simulink model "EEBL_Scenario_01_cs"  (Simulink 7.6)
settings: Solver=ode5  SolverMode=SingleTasking  StartTime=0.0  StopTime=inf  FixedStep=1/100  RelTol=1e-3
PreLoadFcn:
  | check_NUTS_defined;
  | 
  | assignin('base',['model_closed_' bdroot],false);addpath('../includes_V2x');
InitFcn:
  | PreScanExperimentInitFcn(bdroot)
StopFcn:
  | PreScanExperimentStopFcn(bdroot)
undefined symbols (not defined in the file or in its folder): acceleration, actorID, actorType, DiscIntNeverNeededParam, GPS_alt, GPS_lat, GPS_long, intmax, lightBarInUse, messageID, publicVehicleType, rotZ, sireneInUse, trafficLightPriority, turnAdvice, velocity, x_ini_VRML, y_ini_VRML, yawRate, z_ini_VRML
libraries: simulink x58, PreScanSimulinkLibrary x12, simulink_extras x10, PreScanUsefulBlocks x6, simulink_need_slupdate x1
(part 2 of 10)

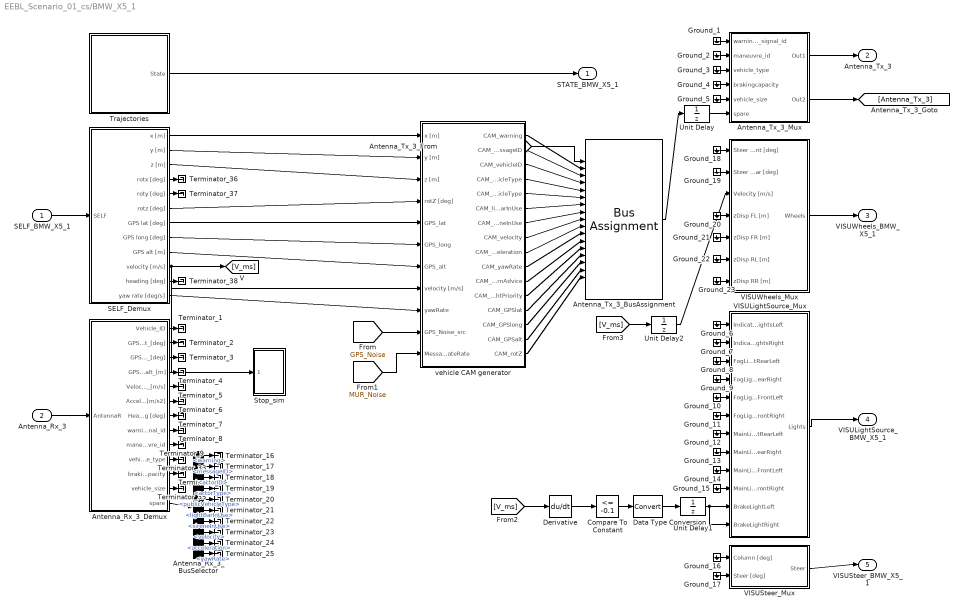
== system EEBL_Scenario_01_cs/BMW_X5_1 ==
  SELF_BMW_X5_1 : Inport  Tag=SELFInport
  Antenna_Rx_3 : Inport  Tag=AntennaRInport  Port=2
  Antenna_Rx_3_BusSelector : BusSelector  Tag=BusAntennaR  OutputSignals=warning,messageID,actorID,actorType,publicVehicleType,lightBarInUse,sireneInUse,velocity,acceleration,yawRate
  Antenna_Rx_3_Demux : Subsystem  Tag=DemuxAntennaR  mask(PreScan Demux Block:){Channel=1}
      settings: DeleteFcn=PreScanBlockDeleteFcn;
      mask Display:
      | fprintf('Channel: %d',Channel)
      | port_label('output', 1, 'Vehicle_ID')
      | port_label('output', 2, 'GPS Pos Lat [deg]')
      | port_label('output', 3, 'GPS Pos Long [deg]')
      | port_label('output', 4, 'GPS Pos Alt [m]')
      | port_label('output', 5, 'Velocity [m/s]')
      | port_label('output', 6, 'Acceleration [m/s2]')
      | port_label('output', 7, 'Heading [deg]')
      | port_label('output', 8, 'Warning signal ID')
      | port_label('output', 9, 'Maneuvre ID')
      | port_label('output', 10, 'Vehicle Type')
      | port_label('output', 11, 'Braking Capacity')
      | port_label('output', 12, 'Vehicle Size')
      | port_label('output', 13, 'Spare')
  Antenna_Tx_3_BusAssignment : BusAssignment  Tag=BusAntennaT  AssignedSignals=warning,messageID,actorID,actorType,publicVehicleType,lightBarInUse,sireneInUse,velocity,acceleration,yawRate,turnAdvice,trafficLightPriority,GPS_lat,GPS_long,GPS_alt,rotZ
  Antenna_Tx_3_Mux : Subsystem  Tag=MuxAntennaT  mask(PreScan Mux Block:){Channel=1, TimeStep=1/100}
      mask prompts: TimeStep "Time Step [s]"
      settings: DeleteFcn=PreScanBlockDeleteFcn;
      mask Display:
      | fprintf('Channel: %d',Channel)
      | port_label('input', 1, 'Warning signal ID')
      | port_label('input', 2, 'Maneuvre ID')
      | port_label('input', 3, 'Vehicle Type')
      | port_label('input', 4, 'Braking Capacity')
      | port_label('input', 5, 'Vehicle Size')
      | port_label('input', 6, 'spare')
  Compare To Constant : simulink/Logic and Bit Operations/Compare To Constant  SystemSampleTime=-1  relop=<=  const=-0.1  LogicOutDataTypeMode=boolean
  Data Type Conversion : DataTypeConversion
  Derivative : Derivative
  Ground_{1..23} (23 alike) : Ground
  SELF_Demux : Subsystem  Tag=DemuxSELF
      settings: DeleteFcn=PreScanBlockDeleteFcn;
      mask Type: PreScan Demux Block:
      mask Display:
      | port_label('output',1,'x [m]')
      | port_label('output',2,'y [m]')
      | port_label('output',3,'z [m]','texmode','on')
      | port_label('output',4,'Rotx [deg]','texmode','on')
      | port_label('output',5,'Roty [deg]','texmode','on')
      | port_label('output',6,'Rotz [deg]','texmode','on')
      | port_label('output',7,'GPS lat [deg]','texmode','on')
      | port_label('output',8,'GPS long [deg]','texmode','on')
      | port_label('output',9,'GPS alt [m]','texmode','on')
      | port_label('output',10,'Velocity [m/s]')
      | port_label('output',11,'Heading [deg]')
      | port_label('output',12,'Yaw rate [deg/s]')
  Stop_sim : Subsystem
  Terminator_{1..9,16..25,33..38} (25 alike) : Terminator
  Trajectories : Subsystem  Tag=Trajectories
      settings: DeleteFcn=PreScanBlockDeleteFcn;
      mask Type: PreScan Source Block: Trajectories
      mask Description:
      | The Trajectory block contains the trajectories defined in the PreScan Experiment Editor. The output of the trajectory block is the (vehicle) State.
      | 
      | For more information, please click Help.
      mask Help: eval('openHelp(312)')
      mask Display: image(imread('Trajectory.png'));
  Unit Delay : UnitDelay  SampleTime=-1
  Unit Delay1 : UnitDelay  SampleTime=-1
  Unit Delay2 : UnitDelay  SampleTime=-1
  VISULightSource_Mux : Subsystem  Tag=MuxLightSource
      settings: DeleteFcn=PreScanBlockDeleteFcn;
      mask Type: PreScan Mux Block:
  VISUSteer_Mux : Subsystem  Tag=MuxSteer
      settings: DeleteFcn=PreScanBlockDeleteFcn;
      mask Type: PreScan Mux Block:
  VISUWheels_Mux : Subsystem  Tag=MuxWheels  mask(PreScan Mux Block:){TimeStep=1/100}
      mask prompts: TimeStep "Auto Assigned: Time Step [s]"
      settings: DeleteFcn=PreScanBlockDeleteFcn;
  vehicle CAM generator : Subsystem
  STATE_BMW_X5_1 : Outport  Tag=StateOutport
  Antenna_Tx_3 : Outport  Tag=AntennaTOutport  Port=2
  VISUWheels_BMW_X5_1 : Outport  Tag=VisuWheelsOutport  Port=3  SampleTime=1/100
  VISULightSource_BMW_X5_1 : Outport  Tag=VisuLightsOutport  Port=4  SampleTime=1/100
  VISUSteer_BMW_X5_1 : Outport  Tag=VisuSteerOutport  Port=5  SampleTime=1/100
  wires:
  [GPS_Noise] -> vehicle CAM generator/10(GPS_Noise_src)
  [MUR_Noise] -> vehicle CAM generator/11(MessageUpdateRate)
  Derivative/1 -> Compare To Constant/1
  Compare To Constant/1 -> Data Type Conversion/1
  Data Type Conversion/1 -> Unit Delay1/1
  [V_ms] -> Derivative/1
  [V_ms] -> Unit Delay2/1
  SELF_BMW_X5_1/1 -> SELF_Demux/1(SELF)
  Antenna_Rx_3_Demux/13(spare) -> Antenna_Rx_3_BusSelector/1
  Antenna_Rx_3/1 -> Antenna_Rx_3_Demux/1(AntennaR)
  Antenna_Tx_3_Mux/2(Out2) -> [Antenna_Tx_3]
  [Antenna_Tx_3] -> Antenna_Tx_3_BusAssignment/1
  Antenna_Tx_3_Mux/1(Out1) -> Antenna_Tx_3/1
  VISUWheels_Mux/1(Wheels) -> VISUWheels_BMW_X5_1/1
  VISULightSource_Mux/1(Lights) -> VISULightSource_BMW_X5_1/1
  VISUSteer_Mux/1(Steer) -> VISUSteer_BMW_X5_1/1
  Trajectories/1(State) -> STATE_BMW_X5_1/1
  SELF_Demux/11(heading [deg]) -> Terminator_38/1
  SELF_Demux/5(roty [deg]) -> Terminator_37/1
  SELF_Demux/4(rotx [deg]) -> Terminator_36/1
  Antenna_Rx_3_Demux/12(vehicle_size) -> Terminator_35/1
  Antenna_Rx_3_Demux/11(brakingcapacity) -> Terminator_34/1
  Antenna_Rx_3_Demux/10(vehicle_type) -> Terminator_33/1
  vehicle CAM generator/16(CAM_rotZ) -> Antenna_Tx_3_BusAssignment/17
  vehicle CAM generator/15(CAM_GPSalt) -> Antenna_Tx_3_BusAssignment/16
  vehicle CAM generator/14(CAM_GPSlong) -> Antenna_Tx_3_BusAssignment/15
  vehicle CAM generator/13(CAM_GPSlat) -> Antenna_Tx_3_BusAssignment/14
  vehicle CAM generator/12(CAM_trafficLightPriority) -> Antenna_Tx_3_BusAssignment/13
  vehicle CAM generator/11(CAM_turnAdvice) -> Antenna_Tx_3_BusAssignment/12
  vehicle CAM generator/10(CAM_yawRate) -> Antenna_Tx_3_BusAssignment/11
  SELF_Demux/12(yaw rate [deg/s]) -> vehicle CAM generator/9(yawRate)
  SELF_Demux/9(GPS alt [m]) -> vehicle CAM generator/7(GPS_alt)
  SELF_Demux/8(GPS long [deg]) -> vehicle CAM generator/6(GPS_long)
  SELF_Demux/7(GPS lat [deg]) -> vehicle CAM generator/5(GPS_lat)
  SELF_Demux/6(rotz [deg]) -> vehicle CAM generator/4(rotZ [deg])
  SELF_Demux/3(z [m]) -> vehicle CAM generator/3(z [m])
  SELF_Demux/2(y [m]) -> vehicle CAM generator/2(y [m])
  SELF_Demux/1(x [m]) -> vehicle CAM generator/1(x [m])
  SELF_Demux/10(velocity [m/s]) -> Stop_sim/1(Velocity), vehicle CAM generator/8(velocity [m/s]), [V_ms]
  vehicle CAM generator/1(CAM_warning) -> Antenna_Tx_3_BusAssignment/2
  vehicle CAM generator/2(CAM_messageID) -> Antenna_Tx_3_BusAssignment/3
  vehicle CAM generator/3(CAM_vehicleID) -> Antenna_Tx_3_BusAssignment/4
  vehicle CAM generator/4(CAM_vehicleType) -> Antenna_Tx_3_BusAssignment/5
  vehicle CAM generator/5(CAM_publicVehicleType) -> Antenna_Tx_3_BusAssignment/6
  vehicle CAM generator/6(CAM_lightBarInUse) -> Antenna_Tx_3_BusAssignment/7
  vehicle CAM generator/7(CAM_sireneInUse) -> Antenna_Tx_3_BusAssignment/8
  vehicle CAM generator/8(CAM_velocity) -> Antenna_Tx_3_BusAssignment/9
  vehicle CAM generator/9(CAM_acceleration) -> Antenna_Tx_3_BusAssignment/10
  Antenna_Rx_3_BusSelector/1 -> Terminator_16/1  "<warning>"
  Antenna_Rx_3_BusSelector/2 -> Terminator_17/1  "<messageID>"
  Antenna_Rx_3_BusSelector/3 -> Terminator_18/1  "<actorID>"
  Antenna_Rx_3_BusSelector/4 -> Terminator_19/1  "<actorType>"
  Antenna_Rx_3_BusSelector/5 -> Terminator_20/1  "<publicVehicleType>"
  Antenna_Rx_3_BusSelector/6 -> Terminator_21/1  "<lightBarInUse>"
  Antenna_Rx_3_BusSelector/7 -> Terminator_22/1  "<sireneInUse>"
  Antenna_Rx_3_BusSelector/8 -> Terminator_23/1  "<velocity>"
  Antenna_Rx_3_BusSelector/9 -> Terminator_24/1  "<acceleration>"
  Antenna_Rx_3_BusSelector/10 -> Terminator_25/1  "<yawRate>"
  Unit Delay/1 -> Antenna_Tx_3_Mux/6(spare)
  Unit Delay1/1 -> VISULightSource_Mux/11(BrakeLightLeft), VISULightSource_Mux/12(BrakeLightRight)
  Unit Delay2/1 -> VISUWheels_Mux/3(Velocity [m/s])
  Antenna_Tx_3_BusAssignment/1 -> Unit Delay/1
  Antenna_Rx_3_Demux/1(Vehicle_ID) -> Terminator_1/1
  Antenna_Rx_3_Demux/2(GPS_pos_lat_[deg]) -> Terminator_2/1
  Antenna_Rx_3_Demux/3(GPS_pos_long_[deg]) -> Terminator_3/1
  Antenna_Rx_3_Demux/4(GPS_pos_alt_[m]) -> Terminator_4/1
  Antenna_Rx_3_Demux/5(Velocity_[m/s]) -> Terminator_5/1
  Antenna_Rx_3_Demux/6(Acceleration_[m/s2]) -> Terminator_6/1
  Antenna_Rx_3_Demux/7(Heading [deg]) -> Terminator_7/1
  Antenna_Rx_3_Demux/8(warning_signal_id) -> Terminator_8/1
  Antenna_Rx_3_Demux/9(maneuvre_id) -> Terminator_9/1
  Ground_1/1 -> Antenna_Tx_3_Mux/1(warning_signal_id)
  Ground_2/1 -> Antenna_Tx_3_Mux/2(maneuvre_id)
  Ground_3/1 -> Antenna_Tx_3_Mux/3(vehicle_type)
  Ground_4/1 -> Antenna_Tx_3_Mux/4(brakingcapacity)
  Ground_5/1 -> Antenna_Tx_3_Mux/5(vehicle_size)
  Ground_6/1 -> VISULightSource_Mux/1(IndicatorLightsLeft)
  Ground_7/1 -> VISULightSource_Mux/2(IndicatorLightsRight)
  Ground_8/1 -> VISULightSource_Mux/3(FogLightRearLeft)
  Ground_9/1 -> VISULightSource_Mux/4(FogLightRearRight)
  Ground_10/1 -> VISULightSource_Mux/5(FogLightFrontLeft)
  Ground_11/1 -> VISULightSource_Mux/6(FogLightFrontRight)
  Ground_12/1 -> VISULightSource_Mux/7(MainLightRearLeft)
  Ground_13/1 -> VISULightSource_Mux/8(MainLightRearRight)
  Ground_14/1 -> VISULightSource_Mux/9(MainLightFrontLeft)
  Ground_15/1 -> VISULightSource_Mux/10(MainLightFrontRight)
  Ground_16/1 -> VISUSteer_Mux/1(Column [deg])
  Ground_17/1 -> VISUSteer_Mux/2(Steer [deg])
  Ground_18/1 -> VISUWheels_Mux/1(Steer Angle Front [deg])
  Ground_19/1 -> VISUWheels_Mux/2(Steer Angle Rear [deg])
  Ground_20/1 -> VISUWheels_Mux/4(zDisp FL [m])
  Ground_21/1 -> VISUWheels_Mux/5(zDisp FR [m])
  Ground_22/1 -> VISUWheels_Mux/6(zDisp RL [m])
  Ground_23/1 -> VISUWheels_Mux/7(zDisp RR [m])

== system EEBL_Scenario_01_cs/CollisionDetection ==
  Selector : Selector  IndexMode=Zero-based  IndexOptions=Starting index (dialog)  Indices=PortIndex  OutputSizes=PortWidth(1)
  retrieve CollisionDetection signal : Subsystem
  U : Outport
  U1 : Outport  Port=2
  wires:
  retrieve CollisionDetection signal/1(Out) -> U1/1
  [SimCoreSensors] -> Selector/1
  Selector/1 -> retrieve CollisionDetection signal/1(In), U/1

== system EEBL_Scenario_01_cs/GetSensors ==
  dummy : Inport
  GetSensors : M-S-Function  FunctionName=GetSensorsBlock  Parameters=TimeStep NrOfSensors
  tag scope: SimCoreSensors=global
  wires:
  GetSensors/1 -> [SimCoreSensors]
  dummy/1 -> GetSensors/1

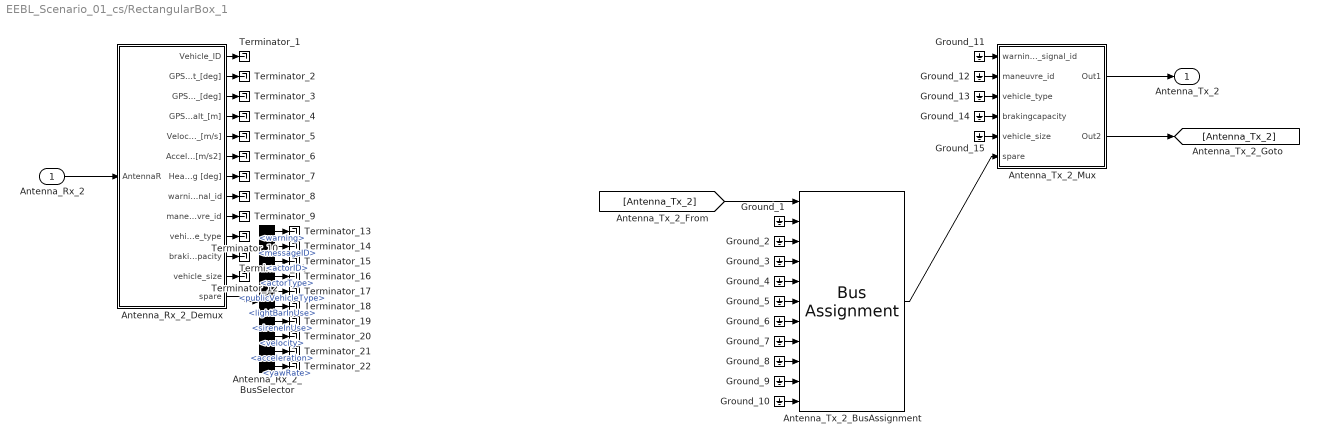
== system EEBL_Scenario_01_cs/RectangularBox_1 ==
  Antenna_Rx_2 : Inport  Tag=AntennaRInport
  Antenna_Rx_2_BusSelector : BusSelector  Tag=BusAntennaR  OutputSignals=warning,messageID,actorID,actorType,publicVehicleType,lightBarInUse,sireneInUse,velocity,acceleration,yawRate
  Antenna_Rx_2_Demux : Subsystem  Tag=DemuxAntennaR  mask(PreScan Demux Block:){Channel=1}
      settings: DeleteFcn=PreScanBlockDeleteFcn;
      mask Display:
      | fprintf('Channel: %d',Channel)
      | port_label('output', 1, 'Vehicle_ID')
      | port_label('output', 2, 'GPS Pos Lat [deg]')
      | port_label('output', 3, 'GPS Pos Long [deg]')
      | port_label('output', 4, 'GPS Pos Alt [m]')
      | port_label('output', 5, 'Velocity [m/s]')
      | port_label('output', 6, 'Acceleration [m/s2]')
      | port_label('output', 7, 'Heading [deg]')
      | port_label('output', 8, 'Warning signal ID')
      | port_label('output', 9, 'Maneuvre ID')
      | port_label('output', 10, 'Vehicle Type')
      | port_label('output', 11, 'Braking Capacity')
      | port_label('output', 12, 'Vehicle Size')
      | port_label('output', 13, 'Spare')
  Antenna_Tx_2_BusAssignment : BusAssignment  Tag=BusAntennaT  AssignedSignals=warning,messageID,actorID,actorType,publicVehicleType,lightBarInUse,sireneInUse,velocity,acceleration,yawRate
  Antenna_Tx_2_Mux : Subsystem  Tag=MuxAntennaT  mask(PreScan Mux Block:){Channel=1, TimeStep=1/100}
      mask prompts: TimeStep "Time Step [s]"
      settings: DeleteFcn=PreScanBlockDeleteFcn;
      mask Display:
      | fprintf('Channel: %d',Channel)
      | port_label('input', 1, 'Warning signal ID')
      | port_label('input', 2, 'Maneuvre ID')
      | port_label('input', 3, 'Vehicle Type')
      | port_label('input', 4, 'Braking Capacity')
      | port_label('input', 5, 'Vehicle Size')
      | port_label('input', 6, 'spare')
  Ground_{1..15} (15 alike) : Ground
  Terminator_{1..22} (22 alike) : Terminator
  Antenna_Tx_2 : Outport  Tag=AntennaTOutport
  wires:
  Antenna_Rx_2_Demux/13(spare) -> Antenna_Rx_2_BusSelector/1
  Antenna_Rx_2/1 -> Antenna_Rx_2_Demux/1(AntennaR)
  Antenna_Tx_2_Mux/2(Out2) -> [Antenna_Tx_2]
  [Antenna_Tx_2] -> Antenna_Tx_2_BusAssignment/1
  Antenna_Tx_2_BusAssignment/1 -> Antenna_Tx_2_Mux/6(spare)
  Antenna_Tx_2_Mux/1(Out1) -> Antenna_Tx_2/1
  Antenna_Rx_2_BusSelector/1 -> Terminator_13/1  "<warning>"
  Antenna_Rx_2_BusSelector/2 -> Terminator_14/1  "<messageID>"
  Antenna_Rx_2_BusSelector/3 -> Terminator_15/1  "<actorID>"
  Antenna_Rx_2_BusSelector/4 -> Terminator_16/1  "<actorType>"
  Antenna_Rx_2_BusSelector/5 -> Terminator_17/1  "<publicVehicleType>"
  Antenna_Rx_2_BusSelector/6 -> Terminator_18/1  "<lightBarInUse>"
  Antenna_Rx_2_BusSelector/7 -> Terminator_19/1  "<sireneInUse>"
  Antenna_Rx_2_BusSelector/8 -> Terminator_20/1  "<velocity>"
  Antenna_Rx_2_BusSelector/9 -> Terminator_21/1  "<acceleration>"
  Antenna_Rx_2_BusSelector/10 -> Terminator_22/1  "<yawRate>"
  Antenna_Rx_2_Demux/1(Vehicle_ID) -> Terminator_1/1
  Antenna_Rx_2_Demux/2(GPS_pos_lat_[deg]) -> Terminator_2/1
  Antenna_Rx_2_Demux/3(GPS_pos_long_[deg]) -> Terminator_3/1
  Antenna_Rx_2_Demux/4(GPS_pos_alt_[m]) -> Terminator_4/1
  Antenna_Rx_2_Demux/5(Velocity_[m/s]) -> Terminator_5/1
  Antenna_Rx_2_Demux/6(Acceleration_[m/s2]) -> Terminator_6/1
  Antenna_Rx_2_Demux/7(Heading [deg]) -> Terminator_7/1
  Antenna_Rx_2_Demux/8(warning_signal_id) -> Terminator_8/1
  Antenna_Rx_2_Demux/9(maneuvre_id) -> Terminator_9/1
  Antenna_Rx_2_Demux/10(vehicle_type) -> Terminator_10/1
  Antenna_Rx_2_Demux/11(brakingcapacity) -> Terminator_11/1
  Antenna_Rx_2_Demux/12(vehicle_size) -> Terminator_12/1
  Ground_1/1 -> Antenna_Tx_2_BusAssignment/2
  Ground_2/1 -> Antenna_Tx_2_BusAssignment/3
  Ground_3/1 -> Antenna_Tx_2_BusAssignment/4
  Ground_4/1 -> Antenna_Tx_2_BusAssignment/5
  Ground_5/1 -> Antenna_Tx_2_BusAssignment/6
  Ground_6/1 -> Antenna_Tx_2_BusAssignment/7
  Ground_7/1 -> Antenna_Tx_2_BusAssignment/8
  Ground_8/1 -> Antenna_Tx_2_BusAssignment/9
  Ground_9/1 -> Antenna_Tx_2_BusAssignment/10
  Ground_10/1 -> Antenna_Tx_2_BusAssignment/11
  Ground_11/1 -> Antenna_Tx_2_Mux/1(warning_signal_id)
  Ground_12/1 -> Antenna_Tx_2_Mux/2(maneuvre_id)
  Ground_13/1 -> Antenna_Tx_2_Mux/3(vehicle_type)
  Ground_14/1 -> Antenna_Tx_2_Mux/4(brakingcapacity)
  Ground_15/1 -> Antenna_Tx_2_Mux/5(vehicle_size)

== system EEBL_Scenario_01_cs/SELF_Audi_A8_1 ==
  Selector : Selector  IndexMode=Zero-based  IndexOptions=Starting index (dialog)  Indices=PortIndex  OutputSizes=PortWidth(1)
  U : Outport
  wires:
  Selector/1 -> U/1
  [SimCoreSensors] -> Selector/1

== system EEBL_Scenario_01_cs/SELF_BMW_X5_1 ==
  Selector : Selector  IndexMode=Zero-based  IndexOptions=Starting index (dialog)  Indices=PortIndex  OutputSizes=PortWidth(1)
  U : Outport
  wires:
  Selector/1 -> U/1
  [SimCoreSensors] -> Selector/1

== system EEBL_Scenario_01_cs/SELF_Sphere_1 ==
  Selector : Selector  IndexMode=Zero-based  IndexOptions=Starting index (dialog)  Indices=PortIndex  OutputSizes=PortWidth(1)
  U : Outport
  wires:
  Selector/1 -> U/1
  [SimCoreSensors] -> Selector/1

== system EEBL_Scenario_01_cs/STATE_Audi_A8_1 ==
  State : Inport  SampleTime=TimeStep
  Acceleration : Subsystem  mask(ToSensorWorld){PortName=Acceleration_Audi_A8_1, PortIndex=6, PortWidth=3, TimeStep=1/100}
      mask prompts: PortName "Port Name [-]"; PortIndex "Index [-]"; PortWidth "Port Dimensions [-]"; TimeStep "Upload Period [s]"
      mask help: Sends signal(s) from Simulink to the Sensor World
      mask Help:
      | Sends signal(s) from Simulink to the Sensor World.
      | 
      | - Port Name [-]: specifies the name of the output terminal of the Simulink block.
      | - Index [-]: specifies the start position in the output vector sent to the Sensor World
      | - Port dimensions [-]: specifies the width (number of scalars) of the output port
      | - Upload period [s]: specifies the upload period (in seconds) of the port.
      mask Display: port_label('input', 1, PortName)
  Demux : Demux  Outputs=5
  Position : Subsystem  mask(ToSensorWorld){PortName=Position_Audi_A8_1, PortIndex=0, PortWidth=3, TimeStep=1/100}
      mask prompts: PortName "Port Name [-]"; PortIndex "Index [-]"; PortWidth "Port Dimensions [-]"; TimeStep "Upload Period [s]"
      mask help: Sends signal(s) from Simulink to the Sensor World
      mask Help:
      | Sends signal(s) from Simulink to the Sensor World.
      | 
      | - Port Name [-]: specifies the name of the output terminal of the Simulink block.
      | - Index [-]: specifies the start position in the output vector sent to the Sensor World
      | - Port dimensions [-]: specifies the width (number of scalars) of the output port
      | - Upload period [s]: specifies the upload period (in seconds) of the port.
      mask Display: port_label('input', 1, PortName)
  RPY : Subsystem  mask(ToSensorWorld){PortName=RPY_Audi_A8_1, PortIndex=9, PortWidth=3, TimeStep=1/100}
      mask prompts: PortName "Port Name [-]"; PortIndex "Index [-]"; PortWidth "Port Dimensions [-]"; TimeStep "Upload Period [s]"
      mask help: Sends signal(s) from Simulink to the Sensor World
      mask Help:
      | Sends signal(s) from Simulink to the Sensor World.
      | 
      | - Port Name [-]: specifies the name of the output terminal of the Simulink block.
      | - Index [-]: specifies the start position in the output vector sent to the Sensor World
      | - Port dimensions [-]: specifies the width (number of scalars) of the output port
      | - Upload period [s]: specifies the upload period (in seconds) of the port.
      mask Display: port_label('input', 1, PortName)
  Velocity : Subsystem  mask(ToSensorWorld){PortName=Velocity_Audi_A8_1, PortIndex=3, PortWidth=3, TimeStep=1/100}
      mask prompts: PortName "Port Name [-]"; PortIndex "Index [-]"; PortWidth "Port Dimensions [-]"; TimeStep "Upload Period [s]"
      mask help: Sends signal(s) from Simulink to the Sensor World
      mask Help:
      | Sends signal(s) from Simulink to the Sensor World.
      | 
      | - Port Name [-]: specifies the name of the output terminal of the Simulink block.
      | - Index [-]: specifies the start position in the output vector sent to the Sensor World
      | - Port dimensions [-]: specifies the width (number of scalars) of the output port
      | - Upload period [s]: specifies the upload period (in seconds) of the port.
      mask Display: port_label('input', 1, PortName)
  iniBODYAngles wrtVEH [rad] : Constant  Value=[Roll0 Pitch0 0]  SampleTime=TimeStep
  iniVEHAngles wrtGLOB [rad] : Constant  Value=[0 0 Yaw0]  SampleTime=TimeStep
  iniVEHposition wrtGLOB [m] : Constant  Value=[x0 y0 z0]  SampleTime=TimeStep
  state2FullState : PreScanSimulinkLibrary/state2FullState  SystemSampleTime=-1
  velRPY : Subsystem  mask(ToSensorWorld){PortName=velRPY_Audi_A8_1, PortIndex=12, PortWidth=3, TimeStep=1/100}
      mask prompts: PortName "Port Name [-]"; PortIndex "Index [-]"; PortWidth "Port Dimensions [-]"; TimeStep "Upload Period [s]"
      mask help: Sends signal(s) from Simulink to the Sensor World
      mask Help:
      | Sends signal(s) from Simulink to the Sensor World.
      | 
      | - Port Name [-]: specifies the name of the output terminal of the Simulink block.
      | - Index [-]: specifies the start position in the output vector sent to the Sensor World
      | - Port dimensions [-]: specifies the width (number of scalars) of the output port
      | - Upload period [s]: specifies the upload period (in seconds) of the port.
      mask Display: port_label('input', 1, PortName)
  wires:
  Demux/5 -> velRPY/1(Y)
  Demux/4 -> RPY/1(Y)
  Demux/3 -> Acceleration/1(Y)
  Demux/2 -> Velocity/1(Y)
  Demux/1 -> Position/1(Y)
  State/1 -> state2FullState/1
  state2FullState/1 -> Demux/1
  iniVEHposition wrtGLOB [m]/1 -> state2FullState/2
  iniBODYAngles wrtVEH [rad]/1 -> state2FullState/3
  iniVEHAngles wrtGLOB [rad]/1 -> state2FullState/4

== system EEBL_Scenario_01_cs/STATE_BMW_X5_1 ==
  State : Inport  SampleTime=TimeStep
  Acceleration : Subsystem  mask(ToSensorWorld){PortName=Acceleration_BMW_X5_1, PortIndex=457, PortWidth=3, TimeStep=1/100}
      mask prompts: PortName "Port Name [-]"; PortIndex "Index [-]"; PortWidth "Port Dimensions [-]"; TimeStep "Upload Period [s]"
      mask help: Sends signal(s) from Simulink to the Sensor World
      mask Help:
      | Sends signal(s) from Simulink to the Sensor World.
      | 
      | - Port Name [-]: specifies the name of the output terminal of the Simulink block.
      | - Index [-]: specifies the start position in the output vector sent to the Sensor World
      | - Port dimensions [-]: specifies the width (number of scalars) of the output port
      | - Upload period [s]: specifies the upload period (in seconds) of the port.
      mask Display: port_label('input', 1, PortName)
  Demux : Demux  Outputs=5
  Position : Subsystem  mask(ToSensorWorld){PortName=Position_BMW_X5_1, PortIndex=451, PortWidth=3, TimeStep=1/100}
      mask prompts: PortName "Port Name [-]"; PortIndex "Index [-]"; PortWidth "Port Dimensions [-]"; TimeStep "Upload Period [s]"
      mask help: Sends signal(s) from Simulink to the Sensor World
      mask Help:
      | Sends signal(s) from Simulink to the Sensor World.
      | 
      | - Port Name [-]: specifies the name of the output terminal of the Simulink block.
      | - Index [-]: specifies the start position in the output vector sent to the Sensor World
      | - Port dimensions [-]: specifies the width (number of scalars) of the output port
      | - Upload period [s]: specifies the upload period (in seconds) of the port.
      mask Display: port_label('input', 1, PortName)
  RPY : Subsystem  mask(ToSensorWorld){PortName=RPY_BMW_X5_1, PortIndex=460, PortWidth=3, TimeStep=1/100}
      mask prompts: PortName "Port Name [-]"; PortIndex "Index [-]"; PortWidth "Port Dimensions [-]"; TimeStep "Upload Period [s]"
      mask help: Sends signal(s) from Simulink to the Sensor World
      mask Help:
      | Sends signal(s) from Simulink to the Sensor World.
      | 
      | - Port Name [-]: specifies the name of the output terminal of the Simulink block.
      | - Index [-]: specifies the start position in the output vector sent to the Sensor World
      | - Port dimensions [-]: specifies the width (number of scalars) of the output port
      | - Upload period [s]: specifies the upload period (in seconds) of the port.
      mask Display: port_label('input', 1, PortName)
  Velocity : Subsystem  mask(ToSensorWorld){PortName=Velocity_BMW_X5_1, PortIndex=454, PortWidth=3, TimeStep=1/100}
      mask prompts: PortName "Port Name [-]"; PortIndex "Index [-]"; PortWidth "Port Dimensions [-]"; TimeStep "Upload Period [s]"
      mask help: Sends signal(s) from Simulink to the Sensor World
      mask Help:
      | Sends signal(s) from Simulink to the Sensor World.
      | 
      | - Port Name [-]: specifies the name of the output terminal of the Simulink block.
      | - Index [-]: specifies the start position in the output vector sent to the Sensor World
      | - Port dimensions [-]: specifies the width (number of scalars) of the output port
      | - Upload period [s]: specifies the upload period (in seconds) of the port.
      mask Display: port_label('input', 1, PortName)
  iniBODYAngles wrtVEH [rad] : Constant  Value=[Roll0 Pitch0 0]  SampleTime=TimeStep
  iniVEHAngles wrtGLOB [rad] : Constant  Value=[0 0 Yaw0]  SampleTime=TimeStep
  iniVEHposition wrtGLOB [m] : Constant  Value=[x0 y0 z0]  SampleTime=TimeStep
  state2FullState : PreScanSimulinkLibrary/state2FullState  SystemSampleTime=-1
  velRPY : Subsystem  mask(ToSensorWorld){PortName=velRPY_BMW_X5_1, PortIndex=463, PortWidth=3, TimeStep=1/100}
      mask prompts: PortName "Port Name [-]"; PortIndex "Index [-]"; PortWidth "Port Dimensions [-]"; TimeStep "Upload Period [s]"
      mask help: Sends signal(s) from Simulink to the Sensor World
      mask Help:
      | Sends signal(s) from Simulink to the Sensor World.
      | 
      | - Port Name [-]: specifies the name of the output terminal of the Simulink block.
      | - Index [-]: specifies the start position in the output vector sent to the Sensor World
      | - Port dimensions [-]: specifies the width (number of scalars) of the output port
      | - Upload period [s]: specifies the upload period (in seconds) of the port.
      mask Display: port_label('input', 1, PortName)
  wires:
  Demux/5 -> velRPY/1(Y)
  Demux/4 -> RPY/1(Y)
  Demux/3 -> Acceleration/1(Y)
  Demux/2 -> Velocity/1(Y)
  Demux/1 -> Position/1(Y)
  State/1 -> state2FullState/1
  state2FullState/1 -> Demux/1
  iniVEHposition wrtGLOB [m]/1 -> state2FullState/2
  iniBODYAngles wrtVEH [rad]/1 -> state2FullState/3
  iniVEHAngles wrtGLOB [rad]/1 -> state2FullState/4

== system EEBL_Scenario_01_cs/STATE_Sphere_1 ==
  State : Inport  SampleTime=TimeStep
  Acceleration : Subsystem  mask(ToSensorWorld){PortName=Acceleration_Sphere_1, PortIndex=905, PortWidth=3, TimeStep=1/100}
      mask prompts: PortName "Port Name [-]"; PortIndex "Index [-]"; PortWidth "Port Dimensions [-]"; TimeStep "Upload Period [s]"
      mask help: Sends signal(s) from Simulink to the Sensor World
      mask Help:
      | Sends signal(s) from Simulink to the Sensor World.
      | 
      | - Port Name [-]: specifies the name of the output terminal of the Simulink block.
      | - Index [-]: specifies the start position in the output vector sent to the Sensor World
      | - Port dimensions [-]: specifies the width (number of scalars) of the output port
      | - Upload period [s]: specifies the upload period (in seconds) of the port.
      mask Display: port_label('input', 1, PortName)
  Demux : Demux  Outputs=5
  Position : Subsystem  mask(ToSensorWorld){PortName=Position_Sphere_1, PortIndex=899, PortWidth=3, TimeStep=1/100}
      mask prompts: PortName "Port Name [-]"; PortIndex "Index [-]"; PortWidth "Port Dimensions [-]"; TimeStep "Upload Period [s]"
      mask help: Sends signal(s) from Simulink to the Sensor World
      mask Help:
      | Sends signal(s) from Simulink to the Sensor World.
      | 
      | - Port Name [-]: specifies the name of the output terminal of the Simulink block.
      | - Index [-]: specifies the start position in the output vector sent to the Sensor World
      | - Port dimensions [-]: specifies the width (number of scalars) of the output port
      | - Upload period [s]: specifies the upload period (in seconds) of the port.
      mask Display: port_label('input', 1, PortName)
  RPY : Subsystem  mask(ToSensorWorld){PortName=RPY_Sphere_1, PortIndex=908, PortWidth=3, TimeStep=1/100}
      mask prompts: PortName "Port Name [-]"; PortIndex "Index [-]"; PortWidth "Port Dimensions [-]"; TimeStep "Upload Period [s]"
      mask help: Sends signal(s) from Simulink to the Sensor World
      mask Help:
      | Sends signal(s) from Simulink to the Sensor World.
      | 
      | - Port Name [-]: specifies the name of the output terminal of the Simulink block.
      | - Index [-]: specifies the start position in the output vector sent to the Sensor World
      | - Port dimensions [-]: specifies the width (number of scalars) of the output port
      | - Upload period [s]: specifies the upload period (in seconds) of the port.
      mask Display: port_label('input', 1, PortName)
  Velocity : Subsystem  mask(ToSensorWorld){PortName=Velocity_Sphere_1, PortIndex=902, PortWidth=3, TimeStep=1/100}
      mask prompts: PortName "Port Name [-]"; PortIndex "Index [-]"; PortWidth "Port Dimensions [-]"; TimeStep "Upload Period [s]"
      mask help: Sends signal(s) from Simulink to the Sensor World
      mask Help:
      | Sends signal(s) from Simulink to the Sensor World.
      | 
      | - Port Name [-]: specifies the name of the output terminal of the Simulink block.
      | - Index [-]: specifies the start position in the output vector sent to the Sensor World
      | - Port dimensions [-]: specifies the width (number of scalars) of the output port
      | - Upload period [s]: specifies the upload period (in seconds) of the port.
      mask Display: port_label('input', 1, PortName)
  iniBODYAngles wrtVEH [rad] : Constant  Value=[Roll0 Pitch0 0]  SampleTime=TimeStep
  iniVEHAngles wrtGLOB [rad] : Constant  Value=[0 0 Yaw0]  SampleTime=TimeStep
  iniVEHposition wrtGLOB [m] : Constant  Value=[x0 y0 z0]  SampleTime=TimeStep
  state2FullState : PreScanSimulinkLibrary/state2FullState  SystemSampleTime=-1
  velRPY : Subsystem  mask(ToSensorWorld){PortName=velRPY_Sphere_1, PortIndex=911, PortWidth=3, TimeStep=1/100}
      mask prompts: PortName "Port Name [-]"; PortIndex "Index [-]"; PortWidth "Port Dimensions [-]"; TimeStep "Upload Period [s]"
      mask help: Sends signal(s) from Simulink to the Sensor World
      mask Help:
      | Sends signal(s) from Simulink to the Sensor World.
      | 
      | - Port Name [-]: specifies the name of the output terminal of the Simulink block.
      | - Index [-]: specifies the start position in the output vector sent to the Sensor World
      | - Port dimensions [-]: specifies the width (number of scalars) of the output port
      | - Upload period [s]: specifies the upload period (in seconds) of the port.
      mask Display: port_label('input', 1, PortName)
  wires:
  Demux/5 -> velRPY/1(Y)
  Demux/4 -> RPY/1(Y)
  Demux/3 -> Acceleration/1(Y)
  Demux/2 -> Velocity/1(Y)
  Demux/1 -> Position/1(Y)
  State/1 -> state2FullState/1
  state2FullState/1 -> Demux/1
  iniVEHposition wrtGLOB [m]/1 -> state2FullState/2
  iniBODYAngles wrtVEH [rad]/1 -> state2FullState/3
  iniVEHAngles wrtGLOB [rad]/1 -> state2FullState/4

== system EEBL_Scenario_01_cs/Scope Collision Detections ==
  In1 : Inport
  Collision Detections : Scope  NumInputPorts=5
      settings: YMin=0~0~0~0~0  YMax=10~10~10~10~10  SaveName=ScopeData2
  Demux2 : Demux  Outputs=5
  wires:
  Demux2/1 -> Collision Detections/1
  Demux2/2 -> Collision Detections/2
  Demux2/3 -> Collision Detections/3
  Demux2/4 -> Collision Detections/4
  Demux2/5 -> Collision Detections/5
  In1/1 -> Demux2/1

== system EEBL_Scenario_01_cs/Scope Collision IDs ==
  In1 : Inport
  Collision IDs : Scope  NumInputPorts=5
      settings: YMin=0~0~0~0~0  YMax=10~10~10~10~10  SaveName=ScopeData2
  Demux2 : Demux  Outputs=5
  wires:
  In1/1 -> Demux2/1
  Demux2/5 -> Collision IDs/5
  Demux2/4 -> Collision IDs/4
  Demux2/3 -> Collision IDs/3
  Demux2/2 -> Collision IDs/2
  Demux2/1 -> Collision IDs/1

== system EEBL_Scenario_01_cs/SetActuators ==
  Bus Creator : BusCreator  Inputs=1
  Data Store Read : DataStoreRead  DataStoreName=SimCoreActuators  SampleTime=TimeStep
  SendActuators : M-S-Function  FunctionName=SendActuatorsBlock  Parameters=TimeStep NrOfActuators
  dummy : Outport
  tag scope: SimCoreInfo=global
  wires:
  Bus Creator/1 -> [SimCoreInfo]  "SimCore"
  SendActuators/2 -> Bus Creator/1  "ComputationTime[s]"
  SendActuators/1 -> dummy/1
  Data Store Read/1 -> SendActuators/1

== system EEBL_Scenario_01_cs/SimCoreInfo ==
  Bus Selector : BusSelector  OutputSignals=ComputationTime[s]
  Time : Scope
      settings: TimeRange=10  YMin=0  YMax=0.5  SaveName=ComputationTime
  wires:
  Bus Selector/1 -> Time/1  "<ComputationTime[s]>"
  [SimCoreInfo] -> Bus Selector/1

== system EEBL_Scenario_01_cs/Sphere_1 ==
  SELF_Sphere_1 : Inport  Tag=SELFInport
  Dynamics_Empty : Subsystem  Tag=Dynamics_Empty
      mask Display: port_label('output', 1, 'State');text(0,0,' Empty\n')
  Gain : Gain  Gain=[1 1 1 1 1 1 0 0 1]
  SELF_Demux : Subsystem  Tag=DemuxSELF
      settings: DeleteFcn=PreScanBlockDeleteFcn;
      mask Type: PreScan Demux Block:
      mask Display:
      | port_label('output',1,'x [m]')
      | port_label('output',2,'y [m]')
      | port_label('output',3,'z [m]','texmode','on')
      | port_label('output',4,'Rotx [deg]','texmode','on')
      | port_label('output',5,'Roty [deg]','texmode','on')
      | port_label('output',6,'Rotz [deg]','texmode','on')
      | port_label('output',7,'GPS lat [deg]','texmode','on')
      | port_label('output',8,'GPS long [deg]','texmode','on')
      | port_label('output',9,'GPS alt [m]','texmode','on')
      | port_label('output',10,'Velocity [m/s]')
      | port_label('output',11,'Heading [deg]')
      | port_label('output',12,'Yaw rate [deg/s]')
  Terminator_{1..13} (13 alike) : Terminator
  STATE_Sphere_1 : Outport  Tag=StateOutport
  wires:
  [human_view] -> Gain/1
  SELF_Sphere_1/1 -> SELF_Demux/1(SELF)
  Gain/1 -> STATE_Sphere_1/1
  Dynamics_Empty/1(State) -> Terminator_1/1
  SELF_Demux/1(x [m]) -> Terminator_2/1
  SELF_Demux/2(y [m]) -> Terminator_3/1
  SELF_Demux/3(z [m]) -> Terminator_4/1
  SELF_Demux/4(rotx [deg]) -> Terminator_5/1
  SELF_Demux/5(roty [deg]) -> Terminator_6/1
  SELF_Demux/6(rotz [deg]) -> Terminator_7/1
  SELF_Demux/7(GPS lat [deg]) -> Terminator_8/1
  SELF_Demux/8(GPS long [deg]) -> Terminator_9/1
  SELF_Demux/9(GPS alt [m]) -> Terminator_10/1
  SELF_Demux/10(velocity [m/s]) -> Terminator_11/1
  SELF_Demux/11(heading [deg]) -> Terminator_12/1
  SELF_Demux/12(yaw rate [deg/s]) -> Terminator_13/1

== system EEBL_Scenario_01_cs/VISULightSource_Audi_A8_1 ==
  Lights : Inport
  Saturation{1..12} (12 alike) : Saturate  UpperLimit=1  LowerLimit=0
  SubDemuxVisuLightSource : Demux  Outputs=12
  conv_BrakeLightLeft : Subsystem
  conv_BrakeLightRight : Subsystem
  conv_FogLightFrontLeft : Subsystem
  conv_FogLightFrontRight : Subsystem
  conv_FogLightRearLeft : Subsystem
  conv_FogLightRearRight : Subsystem
  conv_IndicatorLightsLeft : Subsystem
  conv_IndicatorLightsRight : Subsystem
  conv_MainLightFrontLeft : Subsystem
  conv_MainLightFrontRight : Subsystem
  conv_MainLightRearLeft : Subsystem
  conv_MainLightRearRight : Subsystem
  visu_BrakeLightLeft_0 : Subsystem  mask(ToSensorWorld){PortName=visu_BrakeLightLeft_0, PortIndex=411, PortWidth=16, TimeStep=1/100}
      mask prompts: PortName "Port Name [-]"; PortIndex "Index [-]"; PortWidth "Port Dimensions [-]"; TimeStep "Upload Period [s]"
      mask help: Sends signal(s) from Simulink to the Sensor World
      mask Help:
      | Sends signal(s) from Simulink to the Sensor World.
      | 
      | - Port Name [-]: specifies the name of the output terminal of the Simulink block.
      | - Index [-]: specifies the start position in the output vector sent to the Sensor World
      | - Port dimensions [-]: specifies the width (number of scalars) of the output port
      | - Upload period [s]: specifies the upload period (in seconds) of the port.
      mask Display: port_label('input', 1, PortName)
  visu_BrakeLightRight_0 : Subsystem  mask(ToSensorWorld){PortName=visu_BrakeLightRight_0, PortIndex=427, PortWidth=16, TimeStep=1/100}
      mask prompts: PortName "Port Name [-]"; PortIndex "Index [-]"; PortWidth "Port Dimensions [-]"; TimeStep "Upload Period [s]"
      mask help: Sends signal(s) from Simulink to the Sensor World
      mask Help:
      | Sends signal(s) from Simulink to the Sensor World.
      | 
      | - Port Name [-]: specifies the name of the output terminal of the Simulink block.
      | - Index [-]: specifies the start position in the output vector sent to the Sensor World
      | - Port dimensions [-]: specifies the width (number of scalars) of the output port
      | - Upload period [s]: specifies the upload period (in seconds) of the port.
      mask Display: port_label('input', 1, PortName)
  visu_FogLightFrontLeft_0 : Subsystem  mask(ToSensorWorld){PortName=visu_FogLightFrontLeft_0, PortIndex=315, PortWidth=16, TimeStep=1/100}
      mask prompts: PortName "Port Name [-]"; PortIndex "Index [-]"; PortWidth "Port Dimensions [-]"; TimeStep "Upload Period [s]"
      mask help: Sends signal(s) from Simulink to the Sensor World
      mask Help:
      | Sends signal(s) from Simulink to the Sensor World.
      | 
      | - Port Name [-]: specifies the name of the output terminal of the Simulink block.
      | - Index [-]: specifies the start position in the output vector sent to the Sensor World
      | - Port dimensions [-]: specifies the width (number of scalars) of the output port
      | - Upload period [s]: specifies the upload period (in seconds) of the port.
      mask Display: port_label('input', 1, PortName)
  visu_FogLightFrontRight_0 : Subsystem  mask(ToSensorWorld){PortName=visu_FogLightFrontRight_0, PortIndex=331, PortWidth=16, TimeStep=1/100}
      mask prompts: PortName "Port Name [-]"; PortIndex "Index [-]"; PortWidth "Port Dimensions [-]"; TimeStep "Upload Period [s]"
      mask help: Sends signal(s) from Simulink to the Sensor World
      mask Help:
      | Sends signal(s) from Simulink to the Sensor World.
      | 
      | - Port Name [-]: specifies the name of the output terminal of the Simulink block.
      | - Index [-]: specifies the start position in the output vector sent to the Sensor World
      | - Port dimensions [-]: specifies the width (number of scalars) of the output port
      | - Upload period [s]: specifies the upload period (in seconds) of the port.
      mask Display: port_label('input', 1, PortName)
  visu_FogLightRearLeft_0 : Subsystem  mask(ToSensorWorld){PortName=visu_FogLightRearLeft_0, PortIndex=283, PortWidth=16, TimeStep=1/100}
      mask prompts: PortName "Port Name [-]"; PortIndex "Index [-]"; PortWidth "Port Dimensions [-]"; TimeStep "Upload Period [s]"
      mask help: Sends signal(s) from Simulink to the Sensor World
      mask Help:
      | Sends signal(s) from Simulink to the Sensor World.
      | 
      | - Port Name [-]: specifies the name of the output terminal of the Simulink block.
      | - Index [-]: specifies the start position in the output vector sent to the Sensor World
      | - Port dimensions [-]: specifies the width (number of scalars) of the output port
      | - Upload period [s]: specifies the upload period (in seconds) of the port.
      mask Display: port_label('input', 1, PortName)
  visu_FogLightRearRight_0 : Subsystem  mask(ToSensorWorld){PortName=visu_FogLightRearRight_0, PortIndex=299, PortWidth=16, TimeStep=1/100}
      mask prompts: PortName "Port Name [-]"; PortIndex "Index [-]"; PortWidth "Port Dimensions [-]"; TimeStep "Upload Period [s]"
      mask help: Sends signal(s) from Simulink to the Sensor World
      mask Help:
      | Sends signal(s) from Simulink to the Sensor World.
      | 
      | - Port Name [-]: specifies the name of the output terminal of the Simulink block.
      | - Index [-]: specifies the start position in the output vector sent to the Sensor World
      | - Port dimensions [-]: specifies the width (number of scalars) of the output port
      | - Upload period [s]: specifies the upload period (in seconds) of the port.
      mask Display: port_label('input', 1, PortName)
  visu_IndicatorLightsLeft_0 : Subsystem  mask(ToSensorWorld){PortName=visu_IndicatorLightsLeft_0, PortIndex=251, PortWidth=16, TimeStep=1/100}
      mask prompts: PortName "Port Name [-]"; PortIndex "Index [-]"; PortWidth "Port Dimensions [-]"; TimeStep "Upload Period [s]"
      mask help: Sends signal(s) from Simulink to the Sensor World
      mask Help:
      | Sends signal(s) from Simulink to the Sensor World.
      | 
      | - Port Name [-]: specifies the name of the output terminal of the Simulink block.
      | - Index [-]: specifies the start position in the output vector sent to the Sensor World
      | - Port dimensions [-]: specifies the width (number of scalars) of the output port
      | - Upload period [s]: specifies the upload period (in seconds) of the port.
      mask Display: port_label('input', 1, PortName)
  visu_IndicatorLightsRight_0 : Subsystem  mask(ToSensorWorld){PortName=visu_IndicatorLightsRight_0, PortIndex=267, PortWidth=16, TimeStep=1/100}
      mask prompts: PortName "Port Name [-]"; PortIndex "Index [-]"; PortWidth "Port Dimensions [-]"; TimeStep "Upload Period [s]"
      mask help: Sends signal(s) from Simulink to the Sensor World
      mask Help:
      | Sends signal(s) from Simulink to the Sensor World.
      | 
      | - Port Name [-]: specifies the name of the output terminal of the Simulink block.
      | - Index [-]: specifies the start position in the output vector sent to the Sensor World
      | - Port dimensions [-]: specifies the width (number of scalars) of the output port
      | - Upload period [s]: specifies the upload period (in seconds) of the port.
      mask Display: port_label('input', 1, PortName)
  visu_MainLightFrontLeft_0 : Subsystem  mask(ToSensorWorld){PortName=visu_MainLightFrontLeft_0, PortIndex=379, PortWidth=16, TimeStep=1/100}
      mask prompts: PortName "Port Name [-]"; PortIndex "Index [-]"; PortWidth "Port Dimensions [-]"; TimeStep "Upload Period [s]"
      mask help: Sends signal(s) from Simulink to the Sensor World
      mask Help:
      | Sends signal(s) from Simulink to the Sensor World.
      | 
      | - Port Name [-]: specifies the name of the output terminal of the Simulink block.
      | - Index [-]: specifies the start position in the output vector sent to the Sensor World
      | - Port dimensions [-]: specifies the width (number of scalars) of the output port
      | - Upload period [s]: specifies the upload period (in seconds) of the port.
      mask Display: port_label('input', 1, PortName)
  visu_MainLightFrontRight_0 : Subsystem  mask(ToSensorWorld){PortName=visu_MainLightFrontRight_0, PortIndex=395, PortWidth=16, TimeStep=1/100}
      mask prompts: PortName "Port Name [-]"; PortIndex "Index [-]"; PortWidth "Port Dimensions [-]"; TimeStep "Upload Period [s]"
      mask help: Sends signal(s) from Simulink to the Sensor World
      mask Help:
      | Sends signal(s) from Simulink to the Sensor World.
      | 
      | - Port Name [-]: specifies the name of the output terminal of the Simulink block.
      | - Index [-]: specifies the start position in the output vector sent to the Sensor World
      | - Port dimensions [-]: specifies the width (number of scalars) of the output port
      | - Upload period [s]: specifies the upload period (in seconds) of the port.
      mask Display: port_label('input', 1, PortName)
  visu_MainLightRearLeft_0 : Subsystem  mask(ToSensorWorld){PortName=visu_MainLightRearLeft_0, PortIndex=347, PortWidth=16, TimeStep=1/100}
      mask prompts: PortName "Port Name [-]"; PortIndex "Index [-]"; PortWidth "Port Dimensions [-]"; TimeStep "Upload Period [s]"
      mask help: Sends signal(s) from Simulink to the Sensor World
      mask Help:
      | Sends signal(s) from Simulink to the Sensor World.
      | 
      | - Port Name [-]: specifies the name of the output terminal of the Simulink block.
      | - Index [-]: specifies the start position in the output vector sent to the Sensor World
      | - Port dimensions [-]: specifies the width (number of scalars) of the output port
      | - Upload period [s]: specifies the upload period (in seconds) of the port.
      mask Display: port_label('input', 1, PortName)
  visu_MainLightRearRight_0 : Subsystem  mask(ToSensorWorld){PortName=visu_MainLightRearRight_0, PortIndex=363, PortWidth=16, TimeStep=1/100}
      mask prompts: PortName "Port Name [-]"; PortIndex "Index [-]"; PortWidth "Port Dimensions [-]"; TimeStep "Upload Period [s]"
      mask help: Sends signal(s) from Simulink to the Sensor World
      mask Help:
      | Sends signal(s) from Simulink to the Sensor World.
      | 
      | - Port Name [-]: specifies the name of the output terminal of the Simulink block.
      | - Index [-]: specifies the start position in the output vector sent to the Sensor World
      | - Port dimensions [-]: specifies the width (number of scalars) of the output port
      | - Upload period [s]: specifies the upload period (in seconds) of the port.
      mask Display: port_label('input', 1, PortName)
  wires:
  Lights/1 -> SubDemuxVisuLightSource/1
  SubDemuxVisuLightSource/1 -> Saturation1/1
  Saturation1/1 -> conv_IndicatorLightsLeft/1(on_off)
  conv_IndicatorLightsLeft/1(RGBcolor) -> visu_IndicatorLightsLeft_0/1(Y)
  SubDemuxVisuLightSource/2 -> Saturation2/1
  Saturation2/1 -> conv_IndicatorLightsRight/1(on_off)
  conv_IndicatorLightsRight/1(RGBcolor) -> visu_IndicatorLightsRight_0/1(Y)
  SubDemuxVisuLightSource/3 -> Saturation3/1
  Saturation3/1 -> conv_FogLightRearLeft/1(on_off)
  conv_FogLightRearLeft/1(RGBcolor) -> visu_FogLightRearLeft_0/1(Y)
  SubDemuxVisuLightSource/4 -> Saturation4/1
  Saturation4/1 -> conv_FogLightRearRight/1(on_off)
  conv_FogLightRearRight/1(RGBcolor) -> visu_FogLightRearRight_0/1(Y)
  SubDemuxVisuLightSource/5 -> Saturation5/1
  Saturation5/1 -> conv_FogLightFrontLeft/1(on_off)
  conv_FogLightFrontLeft/1(RGBcolor) -> visu_FogLightFrontLeft_0/1(Y)
  SubDemuxVisuLightSource/6 -> Saturation6/1
  Saturation6/1 -> conv_FogLightFrontRight/1(on_off)
  conv_FogLightFrontRight/1(RGBcolor) -> visu_FogLightFrontRight_0/1(Y)
  SubDemuxVisuLightSource/7 -> Saturation7/1
  Saturation7/1 -> conv_MainLightRearLeft/1(on_off)
  conv_MainLightRearLeft/1(RGBcolor) -> visu_MainLightRearLeft_0/1(Y)
  SubDemuxVisuLightSource/8 -> Saturation8/1
  Saturation8/1 -> conv_MainLightRearRight/1(on_off)
  conv_MainLightRearRight/1(RGBcolor) -> visu_MainLightRearRight_0/1(Y)
  SubDemuxVisuLightSource/9 -> Saturation9/1
  Saturation9/1 -> conv_MainLightFrontLeft/1(on_off)
  conv_MainLightFrontLeft/1(RGBcolor) -> visu_MainLightFrontLeft_0/1(Y)
  SubDemuxVisuLightSource/10 -> Saturation10/1
  Saturation10/1 -> conv_MainLightFrontRight/1(on_off)
  conv_MainLightFrontRight/1(RGBcolor) -> visu_MainLightFrontRight_0/1(Y)
  SubDemuxVisuLightSource/11 -> Saturation11/1
  Saturation11/1 -> conv_BrakeLightLeft/1(on_off)
  conv_BrakeLightLeft/1(RGBcolor) -> visu_BrakeLightLeft_0/1(Y)
  SubDemuxVisuLightSource/12 -> Saturation12/1
  Saturation12/1 -> conv_BrakeLightRight/1(on_off)
  conv_BrakeLightRight/1(RGBcolor) -> visu_BrakeLightRight_0/1(Y)
